simulink model "mdl_positionLoop_3"  (R2022b)
settings: Solver=VariableStepAuto  StartTime=0.0  StopTime=2  RelTol=1e-3
values from neighbouring files (symbols this model uses):
  J = 0.00016    [m2_5_1.m]    (also in m2_5_2.m)
settings Model: Creator=jack  LastModifiedBy=jackyeh

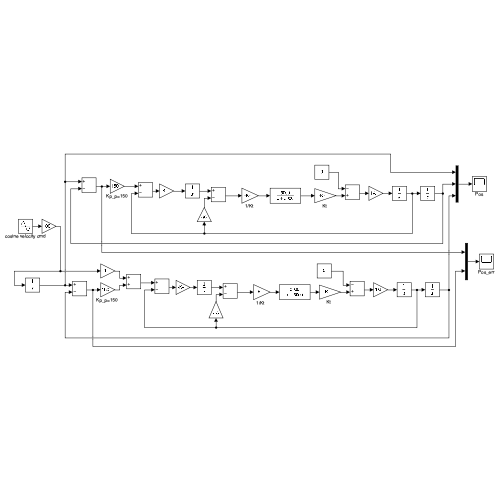
[thumbnail: Simulink's stored preview of the top-level diagram]
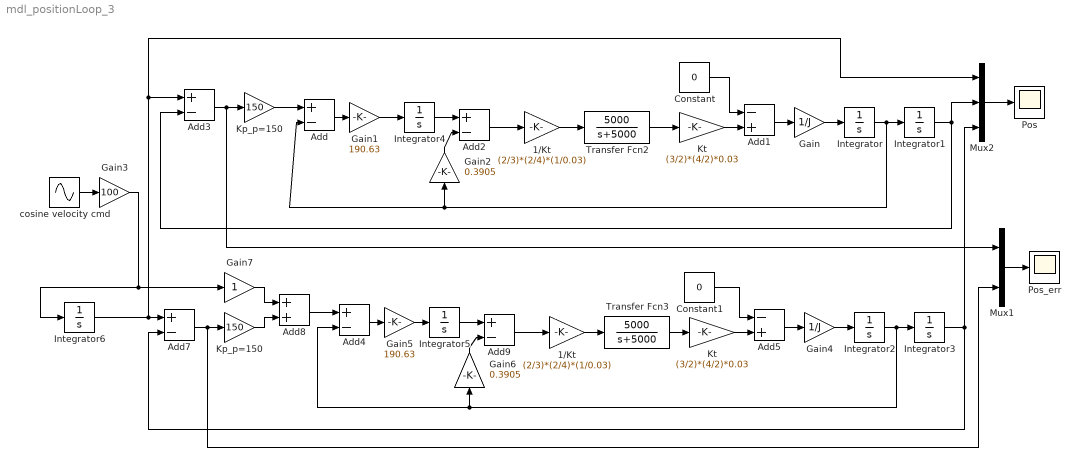
== system mdl_positionLoop_3 ==
  "1/Kt " : Gain  Gain=(2/3)*(2/4)*(1/0.03)
  "1/Kt  " : Gain  Gain=(2/3)*(2/4)*(1/0.03)
  Add{,2..4,7,9} (6 alike) : Sum  Inputs=+-
  Add1 : Sum  Inputs=-+
  Add5 : Sum  Inputs=-+
  Add8 : Sum
  Constant : Constant  Value=0
  Constant1 : Constant  Value=0
  Gain : Gain  Gain=1/J
  Gain1 : Gain  Gain=190.63
  Gain2 : Gain  Gain=0.3905
  Gain3 : Gain  Gain=100
  Gain4 : Gain  Gain=1/J
  Gain5 : Gain  Gain=190.63
  Gain6 : Gain  Gain=0.3905
  Gain7 : Gain
  Integrator{,1..6} (7 alike) : Integrator
  Kp_p=150 : Gain  Gain=150
  "Kp_p=150 " : Gain  Gain=150
  "Kt " : Gain  Gain=(3/2)*(4/2)*0.03
  "Kt  " : Gain  Gain=(3/2)*(4/2)*0.03
  Mux1 : Mux  Inputs=2
  Mux2 : Mux  Inputs=3
  Pos : Scope
  Pos_err : Scope
  Transfer Fcn2 : TransferFcn  Numerator=[5000]  Denominator=[1 5000]
  Transfer Fcn3 : TransferFcn  Numerator=[5000]  Denominator=[1 5000]
  cosine velocity cmd : Sin  Frequency=2*pi*5  Phase=pi/2  SampleTime=0
  wires:
  Gain/1 -> Integrator/1
  Integrator/1 -> Integrator1/1, Gain2/1, Add/2
  Constant/1 -> Add1/1
  Add1/1 -> Gain/1
  Add2/1 -> "1/Kt "/1
  Mux2/1 -> Pos/1
  "1/Kt "/1 -> Transfer Fcn2/1
  "Kt "/1 -> Add1/2
  cosine velocity cmd/1 -> Gain3/1
  Transfer Fcn2/1 -> "Kt "/1
  Add3/1 -> Mux1/1, Kp_p=150/1
  Kp_p=150/1 -> Add/1
  Integrator1/1 -> Mux2/2, Add3/2
  Integrator3/1 -> Mux2/3, Add7/2
  Add7/1 -> Mux1/2, "Kp_p=150 "/1
  Transfer Fcn3/1 -> "Kt  "/1
  "Kt  "/1 -> Add5/2
  "1/Kt  "/1 -> Transfer Fcn3/1
  Add5/1 -> Gain4/1
  Constant1/1 -> Add5/1
  Integrator2/1 -> Add4/2, Gain6/1, Integrator3/1
  Gain4/1 -> Integrator2/1
  "Kp_p=150 "/1 -> Add8/2
  Add8/1 -> Add4/1
  Mux1/1 -> Pos_err/1
  Gain7/1 -> Add8/1
  Add/1 -> Gain1/1
  Gain1/1 -> Integrator4/1
  Integrator4/1 -> Add2/1
  Gain2/1 -> Add2/2
  Gain6/1 -> Add9/2
  Integrator5/1 -> Add9/1
  Gain5/1 -> Integrator5/1
  Add9/1 -> "1/Kt  "/1
  Add4/1 -> Gain5/1
  Gain3/1 -> Integrator6/1, Gain7/1
  Integrator6/1 -> Mux2/1, Add3/1, Add7/1
